simulink model "DriveSystemControl"  (R2023b)
settings: Solver=FixedStepAuto  StartTime=0.0  StopTime=Inf  FixedStep=0.001  RelTol=1e-3
PostLoadFcn:
  | if any(exist('dsrtsu_mdlpostloadfcn', 'file') ~= 0), dsrtsu_mdlpostloadfcn('Execute', bdroot); end
InitFcn:
  | , if any(exist('rtifpga_mdlclblib', 'file') ~= 0), rtifpga_mdlclblib('Init', bdroot); end,
  | , if any(exist('dsmpb_private', 'file') ~= 0), dsmpb_private('dsmpb_mdlclblib', 'Init', bdroot); end,
libraries: dsmpblib x2
(part 10 of 11)

== system DriveSystemControl/Bus Configuration (1) - Out/Manipulation/Virya Controller CAN File 08082024/WIP/CANChannel/PDUs/TCU04/sigMCU5_DriveMode/Feature Switch ==
  Feature Switch : Inport
  Term_sigMCU5_DriveMode Current Countdown Value : Terminator
  Term_sigMCU5_DriveMode Selected Feature : Terminator
  _Feature Switch_ : BusSelector  OutputSignals=sigMCU5_DriveMode Current Countdown Value,sigMCU5_DriveMode Selected Feature
  wires:
  Feature Switch/1 -> _Feature Switch_/1  "Feature Switch"
  _Feature Switch_/1 -> Term_sigMCU5_DriveMode Current Countdown Value/1  "<sigMCU5_DriveMode Current Countdown Value>"
  _Feature Switch_/2 -> Term_sigMCU5_DriveMode Selected Feature/1  "<sigMCU5_DriveMode Selected Feature>"

== system DriveSystemControl/Bus Configuration (1) - Out/Manipulation/Virya Controller CAN File 08082024/WIP/CANChannel/PDUs/TCU04/sigMCU5_Efficiency/Feature Switch ==
  Feature Switch : Inport
  Term_sigMCU5_Efficiency Current Countdown Value : Terminator
  Term_sigMCU5_Efficiency Selected Feature : Terminator
  _Feature Switch_ : BusSelector  OutputSignals=sigMCU5_Efficiency Current Countdown Value,sigMCU5_Efficiency Selected Feature
  wires:
  Feature Switch/1 -> _Feature Switch_/1  "Feature Switch"
  _Feature Switch_/1 -> Term_sigMCU5_Efficiency Current Countdown Value/1  "<sigMCU5_Efficiency Current Countdown Value>"
  _Feature Switch_/2 -> Term_sigMCU5_Efficiency Selected Feature/1  "<sigMCU5_Efficiency Selected Feature>"

== system DriveSystemControl/Bus Configuration (1) - Out/Manipulation/Virya Controller CAN File 08082024/WIP/CANChannel/PDUs/TCU04/sigMCU5_Hillhold/Feature Switch ==
  Feature Switch : Inport
  Term_sigMCU5_Hillhold Current Countdown Value : Terminator
  Term_sigMCU5_Hillhold Selected Feature : Terminator
  _Feature Switch_ : BusSelector  OutputSignals=sigMCU5_Hillhold Current Countdown Value,sigMCU5_Hillhold Selected Feature
  wires:
  Feature Switch/1 -> _Feature Switch_/1  "Feature Switch"
  _Feature Switch_/1 -> Term_sigMCU5_Hillhold Current Countdown Value/1  "<sigMCU5_Hillhold Current Countdown Value>"
  _Feature Switch_/2 -> Term_sigMCU5_Hillhold Selected Feature/1  "<sigMCU5_Hillhold Selected Feature>"

== system DriveSystemControl/Bus Configuration (1) - Out/Manipulation/Virya Controller CAN File 08082024/WIP/CANChannel/PDUs/TCU04/sigMCU5_RegenFlag/Feature Switch ==
  Feature Switch : Inport
  Term_sigMCU5_RegenFlag Current Countdown Value : Terminator
  Term_sigMCU5_RegenFlag Selected Feature : Terminator
  _Feature Switch_ : BusSelector  OutputSignals=sigMCU5_RegenFlag Current Countdown Value,sigMCU5_RegenFlag Selected Feature
  wires:
  Feature Switch/1 -> _Feature Switch_/1  "Feature Switch"
  _Feature Switch_/1 -> Term_sigMCU5_RegenFlag Current Countdown Value/1  "<sigMCU5_RegenFlag Current Countdown Value>"
  _Feature Switch_/2 -> Term_sigMCU5_RegenFlag Selected Feature/1  "<sigMCU5_RegenFlag Selected Feature>"

== system DriveSystemControl/Bus Configuration (1) - Out/Manipulation/Virya Controller CAN File 08082024/WIP/CANChannel/PDUs/TCU04/sigMCU5_Speed/Feature Switch ==
  Feature Switch : Inport
  Term_sigMCU5_Speed Current Countdown Value : Terminator
  Term_sigMCU5_Speed Selected Feature : Terminator
  _Feature Switch_ : BusSelector  OutputSignals=sigMCU5_Speed Current Countdown Value,sigMCU5_Speed Selected Feature
  wires:
  Feature Switch/1 -> _Feature Switch_/1  "Feature Switch"
  _Feature Switch_/1 -> Term_sigMCU5_Speed Current Countdown Value/1  "<sigMCU5_Speed Current Countdown Value>"
  _Feature Switch_/2 -> Term_sigMCU5_Speed Selected Feature/1  "<sigMCU5_Speed Selected Feature>"

== system DriveSystemControl/Bus Configuration (1) - Out/Manipulation/Virya Controller CAN File 08082024/WIP/CANChannel/PDUs/TCU05/sigMCU6_Odometer/Feature Switch ==
  Feature Switch : Inport
  Term_sigMCU6_Odometer Current Countdown Value : Terminator
  Term_sigMCU6_Odometer Selected Feature : Terminator
  _Feature Switch_ : BusSelector  OutputSignals=sigMCU6_Odometer Current Countdown Value,sigMCU6_Odometer Selected Feature
  wires:
  Feature Switch/1 -> _Feature Switch_/1  "Feature Switch"
  _Feature Switch_/1 -> Term_sigMCU6_Odometer Current Countdown Value/1  "<sigMCU6_Odometer Current Countdown Value>"
  _Feature Switch_/2 -> Term_sigMCU6_Odometer Selected Feature/1  "<sigMCU6_Odometer Selected Feature>"

== system DriveSystemControl/Bus Configuration (1) - Out/Simulated ECUs/Virya Controller CAN File 08082024/BMS/RX/PDUs/TCU04/sigMCU5_DriveMode/ISignal Value ==
  ISignal Value : Inport
  Term_sigMCU5_DriveMode Value : Terminator
  _ISignal Value_ : BusSelector  OutputSignals=sigMCU5_DriveMode Value
  wires:
  ISignal Value/1 -> _ISignal Value_/1  "ISignal Value"
  _ISignal Value_/1 -> Term_sigMCU5_DriveMode Value/1  "<sigMCU5_DriveMode Value>"

== system DriveSystemControl/Bus Configuration (1) - Out/Simulated ECUs/Virya Controller CAN File 08082024/BMS/RX/PDUs/TCU04/sigMCU5_Efficiency/ISignal Value ==
  ISignal Value : Inport
  Term_sigMCU5_Efficiency Value : Terminator
  _ISignal Value_ : BusSelector  OutputSignals=sigMCU5_Efficiency Value
  wires:
  ISignal Value/1 -> _ISignal Value_/1  "ISignal Value"
  _ISignal Value_/1 -> Term_sigMCU5_Efficiency Value/1  "<sigMCU5_Efficiency Value>"

== system DriveSystemControl/Bus Configuration (1) - Out/Simulated ECUs/Virya Controller CAN File 08082024/BMS/RX/PDUs/TCU04/sigMCU5_Hillhold/ISignal Value ==
  ISignal Value : Inport
  Term_sigMCU5_Hillhold Value : Terminator
  _ISignal Value_ : BusSelector  OutputSignals=sigMCU5_Hillhold Value
  wires:
  ISignal Value/1 -> _ISignal Value_/1  "ISignal Value"
  _ISignal Value_/1 -> Term_sigMCU5_Hillhold Value/1  "<sigMCU5_Hillhold Value>"

== system DriveSystemControl/Bus Configuration (1) - Out/Simulated ECUs/Virya Controller CAN File 08082024/BMS/RX/PDUs/TCU04/sigMCU5_RegenFlag/ISignal Value ==
  ISignal Value : Inport
  Term_sigMCU5_RegenFlag Value : Terminator
  _ISignal Value_ : BusSelector  OutputSignals=sigMCU5_RegenFlag Value
  wires:
  ISignal Value/1 -> _ISignal Value_/1  "ISignal Value"
  _ISignal Value_/1 -> Term_sigMCU5_RegenFlag Value/1  "<sigMCU5_RegenFlag Value>"

== system DriveSystemControl/Bus Configuration (1) - Out/Simulated ECUs/Virya Controller CAN File 08082024/BMS/RX/PDUs/TCU04/sigMCU5_Speed/ISignal Value ==
  ISignal Value : Inport
  Term_sigMCU5_Speed Value : Terminator
  _ISignal Value_ : BusSelector  OutputSignals=sigMCU5_Speed Value
  wires:
  ISignal Value/1 -> _ISignal Value_/1  "ISignal Value"
  _ISignal Value_/1 -> Term_sigMCU5_Speed Value/1  "<sigMCU5_Speed Value>"

== system DriveSystemControl/Bus Configuration (1) - Out/Simulated ECUs/Virya Controller CAN File 08082024/IPC/RX/PDUs/BMS01/sigBatteryMalfunctionLight/ISignal Value ==
  ISignal Value : Inport
  Term_sigBatteryMalfunctionLight Value : Terminator
  _ISignal Value_ : BusSelector  OutputSignals=sigBatteryMalfunctionLight Value
  wires:
  ISignal Value/1 -> _ISignal Value_/1  "ISignal Value"
  _ISignal Value_/1 -> Term_sigBatteryMalfunctionLight Value/1  "<sigBatteryMalfunctionLight Value>"

== system DriveSystemControl/Bus Configuration (1) - Out/Simulated ECUs/Virya Controller CAN File 08082024/IPC/RX/PDUs/BMS01/sigKeyOnIndicator/ISignal Value ==
  ISignal Value : Inport
  Term_sigKeyOnIndicator Value : Terminator
  _ISignal Value_ : BusSelector  OutputSignals=sigKeyOnIndicator Value
  wires:
  ISignal Value/1 -> _ISignal Value_/1  "ISignal Value"
  _ISignal Value_/1 -> Term_sigKeyOnIndicator Value/1  "<sigKeyOnIndicator Value>"

== system DriveSystemControl/Bus Configuration (1) - Out/Simulated ECUs/Virya Controller CAN File 08082024/IPC/RX/PDUs/BMS01/sigStateOfCharge/ISignal Value ==
  ISignal Value : Inport
  Term_sigStateOfCharge Value : Terminator
  _ISignal Value_ : BusSelector  OutputSignals=sigStateOfCharge Value
  wires:
  ISignal Value/1 -> _ISignal Value_/1  "ISignal Value"
  _ISignal Value_/1 -> Term_sigStateOfCharge Value/1  "<sigStateOfCharge Value>"

== system DriveSystemControl/Bus Configuration (1) - Out/Simulated ECUs/Virya Controller CAN File 08082024/IPC/RX/PDUs/TCU01/sigBrake/ISignal Value ==
  ISignal Value : Inport
  Term_sigBrake Value : Terminator
  _ISignal Value_ : BusSelector  OutputSignals=sigBrake Value
  wires:
  ISignal Value/1 -> _ISignal Value_/1  "ISignal Value"
  _ISignal Value_/1 -> Term_sigBrake Value/1  "<sigBrake Value>"

== system DriveSystemControl/Bus Configuration (1) - Out/Simulated ECUs/Virya Controller CAN File 08082024/IPC/RX/PDUs/TCU01/sigControllerTemperature/ISignal Value ==
  ISignal Value : Inport
  Term_sigControllerTemperature Value : Terminator
  _ISignal Value_ : BusSelector  OutputSignals=sigControllerTemperature Value
  wires:
  ISignal Value/1 -> _ISignal Value_/1  "ISignal Value"
  _ISignal Value_/1 -> Term_sigControllerTemperature Value/1  "<sigControllerTemperature Value>"

== system DriveSystemControl/Bus Configuration (1) - Out/Simulated ECUs/Virya Controller CAN File 08082024/IPC/RX/PDUs/TCU01/sigDriveMode/ISignal Value ==
  ISignal Value : Inport
  Term_sigDriveMode Value : Terminator
  _ISignal Value_ : BusSelector  OutputSignals=sigDriveMode Value
  wires:
  ISignal Value/1 -> _ISignal Value_/1  "ISignal Value"
  _ISignal Value_/1 -> Term_sigDriveMode Value/1  "<sigDriveMode Value>"

== system DriveSystemControl/Bus Configuration (1) - Out/Simulated ECUs/Virya Controller CAN File 08082024/IPC/RX/PDUs/TCU01/sigMotorTemperature/ISignal Value ==
  ISignal Value : Inport
  Term_sigMotorTemperature Value : Terminator
  _ISignal Value_ : BusSelector  OutputSignals=sigMotorTemperature Value
  wires:
  ISignal Value/1 -> _ISignal Value_/1  "ISignal Value"
  _ISignal Value_/1 -> Term_sigMotorTemperature Value/1  "<sigMotorTemperature Value>"

== system DriveSystemControl/Bus Configuration (1) - Out/Simulated ECUs/Virya Controller CAN File 08082024/IPC/RX/PDUs/TCU01/sigRMSCurrent/ISignal Value ==
  ISignal Value : Inport
  Term_sigRMSCurrent Value : Terminator
  _ISignal Value_ : BusSelector  OutputSignals=sigRMSCurrent Value
  wires:
  ISignal Value/1 -> _ISignal Value_/1  "ISignal Value"
  _ISignal Value_/1 -> Term_sigRMSCurrent Value/1  "<sigRMSCurrent Value>"

== system DriveSystemControl/Bus Configuration (1) - Out/Simulated ECUs/Virya Controller CAN File 08082024/IPC/RX/PDUs/TCU01/sigSpeed/ISignal Value ==
  ISignal Value : Inport
  Term_sigSpeed Value : Terminator
  _ISignal Value_ : BusSelector  OutputSignals=sigSpeed Value
  wires:
  ISignal Value/1 -> _ISignal Value_/1  "ISignal Value"
  _ISignal Value_/1 -> Term_sigSpeed Value/1  "<sigSpeed Value>"

== system DriveSystemControl/Bus Configuration (1) - Out/Simulated ECUs/Virya Controller CAN File 08082024/IPC/RX/PDUs/TCU01/sigThrottle/ISignal Value ==
  ISignal Value : Inport
  Term_sigThrottle Value : Terminator
  _ISignal Value_ : BusSelector  OutputSignals=sigThrottle Value
  wires:
  ISignal Value/1 -> _ISignal Value_/1  "ISignal Value"
  _ISignal Value_/1 -> Term_sigThrottle Value/1  "<sigThrottle Value>"

== system DriveSystemControl/Bus Configuration (1) - Out/Simulated ECUs/Virya Controller CAN File 08082024/IPC/RX/PDUs/TCU03/Controller_CompleteFaults/ISignal Value ==
  ISignal Value : Inport
  Term_Controller_CompleteFaults Value : Terminator
  _ISignal Value_ : BusSelector  OutputSignals=Controller_CompleteFaults Value
  wires:
  ISignal Value/1 -> _ISignal Value_/1  "ISignal Value"
  _ISignal Value_/1 -> Term_Controller_CompleteFaults Value/1  "<Controller_CompleteFaults Value>"

== system DriveSystemControl/Bus Configuration (1) - Out/Simulated ECUs/Virya Controller CAN File 08082024/IPC/RX/PDUs/TCU03/sig5VSupplyFailure/ISignal Value ==
  ISignal Value : Inport
  Term_sig5VSupplyFailure Value : Terminator
  _ISignal Value_ : BusSelector  OutputSignals=sig5VSupplyFailure Value
  wires:
  ISignal Value/1 -> _ISignal Value_/1  "ISignal Value"
  _ISignal Value_/1 -> Term_sig5VSupplyFailure Value/1  "<sig5VSupplyFailure Value>"

== system DriveSystemControl/Bus Configuration (1) - Out/Simulated ECUs/Virya Controller CAN File 08082024/IPC/RX/PDUs/TCU03/sigBPosOvervoltageCutback/ISignal Value ==
  ISignal Value : Inport
  Term_sigBPosOvervoltageCutback Value : Terminator
  _ISignal Value_ : BusSelector  OutputSignals=sigBPosOvervoltageCutback Value
  wires:
  ISignal Value/1 -> _ISignal Value_/1  "ISignal Value"
  _ISignal Value_/1 -> Term_sigBPosOvervoltageCutback Value/1  "<sigBPosOvervoltageCutback Value>"

== system DriveSystemControl/Bus Configuration (1) - Out/Simulated ECUs/Virya Controller CAN File 08082024/IPC/RX/PDUs/TCU03/sigBPosUndervoltageCutback/ISignal Value ==
  ISignal Value : Inport
  Term_sigBPosUndervoltageCutback Value : Terminator
  _ISignal Value_ : BusSelector  OutputSignals=sigBPosUndervoltageCutback Value
  wires:
  ISignal Value/1 -> _ISignal Value_/1  "ISignal Value"
  _ISignal Value_/1 -> Term_sigBPosUndervoltageCutback Value/1  "<sigBPosUndervoltageCutback Value>"

== system DriveSystemControl/Bus Configuration (1) - Out/Simulated ECUs/Virya Controller CAN File 08082024/IPC/RX/PDUs/TCU03/sigBadCalibration/ISignal Value ==
  ISignal Value : Inport
  Term_sigBadCalibration Value : Terminator
  _ISignal Value_ : BusSelector  OutputSignals=sigBadCalibration Value
  wires:
  ISignal Value/1 -> _ISignal Value_/1  "ISignal Value"
  _ISignal Value_/1 -> Term_sigBadCalibration Value/1  "<sigBadCalibration Value>"

== system DriveSystemControl/Bus Configuration (1) - Out/Simulated ECUs/Virya Controller CAN File 08082024/IPC/RX/PDUs/TCU03/sigBrakeWiperHigh/ISignal Value ==
  ISignal Value : Inport
  Term_sigBrakeWiperHigh Value : Terminator
  _ISignal Value_ : BusSelector  OutputSignals=sigBrakeWiperHigh Value
  wires:
  ISignal Value/1 -> _ISignal Value_/1  "ISignal Value"
  _ISignal Value_/1 -> Term_sigBrakeWiperHigh Value/1  "<sigBrakeWiperHigh Value>"

== system DriveSystemControl/Bus Configuration (1) - Out/Simulated ECUs/Virya Controller CAN File 08082024/IPC/RX/PDUs/TCU03/sigBrakeWiperLow/ISignal Value ==
  ISignal Value : Inport
  Term_sigBrakeWiperLow Value : Terminator
  _ISignal Value_ : BusSelector  OutputSignals=sigBrakeWiperLow Value
  wires:
  ISignal Value/1 -> _ISignal Value_/1  "ISignal Value"
  _ISignal Value_/1 -> Term_sigBrakeWiperLow Value/1  "<sigBrakeWiperLow Value>"

== system DriveSystemControl/Bus Configuration (1) - Out/Simulated ECUs/Virya Controller CAN File 08082024/IPC/RX/PDUs/TCU03/sigCoil2DriverOpenShort/ISignal Value ==
  ISignal Value : Inport
  Term_sigCoil2DriverOpenShort Value : Terminator
  _ISignal Value_ : BusSelector  OutputSignals=sigCoil2DriverOpenShort Value
  wires:
  ISignal Value/1 -> _ISignal Value_/1  "ISignal Value"
  _ISignal Value_/1 -> Term_sigCoil2DriverOpenShort Value/1  "<sigCoil2DriverOpenShort Value>"

== system DriveSystemControl/Bus Configuration (1) - Out/Simulated ECUs/Virya Controller CAN File 08082024/IPC/RX/PDUs/TCU03/sigCoil3DriverOpenShort/ISignal Value ==
  ISignal Value : Inport
  Term_sigCoil3DriverOpenShort Value : Terminator
  _ISignal Value_ : BusSelector  OutputSignals=sigCoil3DriverOpenShort Value
  wires:
  ISignal Value/1 -> _ISignal Value_/1  "ISignal Value"
  _ISignal Value_/1 -> Term_sigCoil3DriverOpenShort Value/1  "<sigCoil3DriverOpenShort Value>"

== system DriveSystemControl/Bus Configuration (1) - Out/Simulated ECUs/Virya Controller CAN File 08082024/IPC/RX/PDUs/TCU03/sigCoil4DriverOpenShort/ISignal Value ==
  ISignal Value : Inport
  Term_sigCoil4DriverOpenShort Value : Terminator
  _ISignal Value_ : BusSelector  OutputSignals=sigCoil4DriverOpenShort Value
  wires:
  ISignal Value/1 -> _ISignal Value_/1  "ISignal Value"
  _ISignal Value_/1 -> Term_sigCoil4DriverOpenShort Value/1  "<sigCoil4DriverOpenShort Value>"

== system DriveSystemControl/Bus Configuration (1) - Out/Simulated ECUs/Virya Controller CAN File 08082024/IPC/RX/PDUs/TCU03/sigControllerCommonFault/ISignal Value ==
  ISignal Value : Inport
  Term_sigControllerCommonFault Value : Terminator
  _ISignal Value_ : BusSelector  OutputSignals=sigControllerCommonFault Value
  wires:
  ISignal Value/1 -> _ISignal Value_/1  "ISignal Value"
  _ISignal Value_/1 -> Term_sigControllerCommonFault Value/1  "<sigControllerCommonFault Value>"

== system DriveSystemControl/Bus Configuration (1) - Out/Simulated ECUs/Virya Controller CAN File 08082024/IPC/RX/PDUs/TCU03/sigControllerOverCurrent/ISignal Value ==
  ISignal Value : Inport
  Term_sigControllerOverCurrent Value : Terminator
  _ISignal Value_ : BusSelector  OutputSignals=sigControllerOverCurrent Value
  wires:
  ISignal Value/1 -> _ISignal Value_/1  "ISignal Value"
  _ISignal Value_/1 -> Term_sigControllerOverCurrent Value/1  "<sigControllerOverCurrent Value>"

== system DriveSystemControl/Bus Configuration (1) - Out/Simulated ECUs/Virya Controller CAN File 08082024/IPC/RX/PDUs/TCU03/sigControllerOvertempCutback/ISignal Value ==
  ISignal Value : Inport
  Term_sigControllerOvertempCutback Value : Terminator
  _ISignal Value_ : BusSelector  OutputSignals=sigControllerOvertempCutback Value
  wires:
  ISignal Value/1 -> _ISignal Value_/1  "ISignal Value"
  _ISignal Value_/1 -> Term_sigControllerOvertempCutback Value/1  "<sigControllerOvertempCutback Value>"

== system DriveSystemControl/Bus Configuration (1) - Out/Simulated ECUs/Virya Controller CAN File 08082024/IPC/RX/PDUs/TCU03/sigControllerSevereOvertemp/ISignal Value ==
  ISignal Value : Inport
  Term_sigControllerSevereOvertemp Value : Terminator
  _ISignal Value_ : BusSelector  OutputSignals=sigControllerSevereOvertemp Value
  wires:
  ISignal Value/1 -> _ISignal Value_/1  "ISignal Value"
  _ISignal Value_/1 -> Term_sigControllerSevereOvertemp Value/1  "<sigControllerSevereOvertemp Value>"

== system DriveSystemControl/Bus Configuration (1) - Out/Simulated ECUs/Virya Controller CAN File 08082024/IPC/RX/PDUs/TCU03/sigControllerSevereUndertemp/ISignal Value ==
  ISignal Value : Inport
  Term_sigControllerSevereUndertemp Value : Terminator
  _ISignal Value_ : BusSelector  OutputSignals=sigControllerSevereUndertemp Value
  wires:
  ISignal Value/1 -> _ISignal Value_/1  "ISignal Value"
  _ISignal Value_/1 -> Term_sigControllerSevereUndertemp Value/1  "<sigControllerSevereUndertemp Value>"

== system DriveSystemControl/Bus Configuration (1) - Out/Simulated ECUs/Virya Controller CAN File 08082024/IPC/RX/PDUs/TCU03/sigCurrentSensorFault/ISignal Value ==
  ISignal Value : Inport
  Term_sigCurrentSensorFault Value : Terminator
  _ISignal Value_ : BusSelector  OutputSignals=sigCurrentSensorFault Value
  wires:
  ISignal Value/1 -> _ISignal Value_/1  "ISignal Value"
  _ISignal Value_/1 -> Term_sigCurrentSensorFault Value/1  "<sigCurrentSensorFault Value>"

== system DriveSystemControl/Bus Configuration (1) - Out/Simulated ECUs/Virya Controller CAN File 08082024/IPC/RX/PDUs/TCU03/sigEEPROMFailure/ISignal Value ==
  ISignal Value : Inport
  Term_sigEEPROMFailure Value : Terminator
  _ISignal Value_ : BusSelector  OutputSignals=sigEEPROMFailure Value
  wires:
  ISignal Value/1 -> _ISignal Value_/1  "ISignal Value"
  _ISignal Value_/1 -> Term_sigEEPROMFailure Value/1  "<sigEEPROMFailure Value>"

== system DriveSystemControl/Bus Configuration (1) - Out/Simulated ECUs/Virya Controller CAN File 08082024/IPC/RX/PDUs/TCU03/sigHighPedalDisable/ISignal Value ==
  ISignal Value : Inport
  Term_sigHighPedalDisable Value : Terminator
  _ISignal Value_ : BusSelector  OutputSignals=sigHighPedalDisable Value
  wires:
  ISignal Value/1 -> _ISignal Value_/1  "ISignal Value"
  _ISignal Value_/1 -> Term_sigHighPedalDisable Value/1  "<sigHighPedalDisable Value>"

== system DriveSystemControl/Bus Configuration (1) - Out/Simulated ECUs/Virya Controller CAN File 08082024/IPC/RX/PDUs/TCU03/sigInsulationResistanceLow/ISignal Value ==
  ISignal Value : Inport
  Term_sigInsulationResistanceLow Value : Terminator
  _ISignal Value_ : BusSelector  OutputSignals=sigInsulationResistanceLow Value
  wires:
  ISignal Value/1 -> _ISignal Value_/1  "ISignal Value"
  _ISignal Value_/1 -> Term_sigInsulationResistanceLow Value/1  "<sigInsulationResistanceLow Value>"

== system DriveSystemControl/Bus Configuration (1) - Out/Simulated ECUs/Virya Controller CAN File 08082024/IPC/RX/PDUs/TCU03/sigMainContactorWelded/ISignal Value ==
  ISignal Value : Inport
  Term_sigMainContactorWelded Value : Terminator
  _ISignal Value_ : BusSelector  OutputSignals=sigMainContactorWelded Value
  wires:
  ISignal Value/1 -> _ISignal Value_/1  "ISignal Value"
  _ISignal Value_/1 -> Term_sigMainContactorWelded Value/1  "<sigMainContactorWelded Value>"

== system DriveSystemControl/Bus Configuration (1) - Out/Simulated ECUs/Virya Controller CAN File 08082024/IPC/RX/PDUs/TCU03/sigMainContactordidnotClose/ISignal Value ==
  ISignal Value : Inport
  Term_sigMainContactordidnotClose Value : Terminator
  _ISignal Value_ : BusSelector  OutputSignals=sigMainContactordidnotClose Value
  wires:
  ISignal Value/1 -> _ISignal Value_/1  "ISignal Value"
  _ISignal Value_/1 -> Term_sigMainContactordidnotClose Value/1  "<sigMainContactordidnotClose Value>"

== system DriveSystemControl/Bus Configuration (1) - Out/Simulated ECUs/Virya Controller CAN File 08082024/IPC/RX/PDUs/TCU03/sigMainOpenShort/ISignal Value ==
  ISignal Value : Inport
  Term_sigMainOpenShort Value : Terminator
  _ISignal Value_ : BusSelector  OutputSignals=sigMainOpenShort Value
  wires:
  ISignal Value/1 -> _ISignal Value_/1  "ISignal Value"
  _ISignal Value_/1 -> Term_sigMainOpenShort Value/1  "<sigMainOpenShort Value>"

== system DriveSystemControl/Bus Configuration (1) - Out/Simulated ECUs/Virya Controller CAN File 08082024/IPC/RX/PDUs/TCU03/sigMotorCharacterization/ISignal Value ==
  ISignal Value : Inport
  Term_sigMotorCharacterization Value : Terminator
  _ISignal Value_ : BusSelector  OutputSignals=sigMotorCharacterization Value
  wires:
  ISignal Value/1 -> _ISignal Value_/1  "ISignal Value"
  _ISignal Value_/1 -> Term_sigMotorCharacterization Value/1  "<sigMotorCharacterization Value>"

== system DriveSystemControl/Bus Configuration (1) - Out/Simulated ECUs/Virya Controller CAN File 08082024/IPC/RX/PDUs/TCU03/sigMotorPhaseOpen/ISignal Value ==
  ISignal Value : Inport
  Term_sigMotorPhaseOpen Value : Terminator
  _ISignal Value_ : BusSelector  OutputSignals=sigMotorPhaseOpen Value
  wires:
  ISignal Value/1 -> _ISignal Value_/1  "ISignal Value"
  _ISignal Value_/1 -> Term_sigMotorPhaseOpen Value/1  "<sigMotorPhaseOpen Value>"

== system DriveSystemControl/Bus Configuration (1) - Out/Simulated ECUs/Virya Controller CAN File 08082024/IPC/RX/PDUs/TCU03/sigMotorTempHotCutback/ISignal Value ==
  ISignal Value : Inport
  Term_sigMotorTempHotCutback Value : Terminator
  _ISignal Value_ : BusSelector  OutputSignals=sigMotorTempHotCutback Value
  wires:
  ISignal Value/1 -> _ISignal Value_/1  "ISignal Value"
  _ISignal Value_/1 -> Term_sigMotorTempHotCutback Value/1  "<sigMotorTempHotCutback Value>"

== system DriveSystemControl/Bus Configuration (1) - Out/Simulated ECUs/Virya Controller CAN File 08082024/IPC/RX/PDUs/TCU03/sigMotorTempSensorFault/ISignal Value ==
  ISignal Value : Inport
  Term_sigMotorTempSensorFault Value : Terminator
  _ISignal Value_ : BusSelector  OutputSignals=sigMotorTempSensorFault Value
  wires:
  ISignal Value/1 -> _ISignal Value_/1  "ISignal Value"
  _ISignal Value_/1 -> Term_sigMotorTempSensorFault Value/1  "<sigMotorTempSensorFault Value>"

== system DriveSystemControl/Bus Configuration (1) - Out/Simulated ECUs/Virya Controller CAN File 08082024/IPC/RX/PDUs/TCU03/sigOEM_BatterySTOPSignal/ISignal Value ==
  ISignal Value : Inport
  Term_sigOEM_BatterySTOPSignal Value : Terminator
  _ISignal Value_ : BusSelector  OutputSignals=sigOEM_BatterySTOPSignal Value
  wires:
  ISignal Value/1 -> _ISignal Value_/1  "ISignal Value"
  _ISignal Value_/1 -> Term_sigOEM_BatterySTOPSignal Value/1  "<sigOEM_BatterySTOPSignal Value>"

== system DriveSystemControl/Bus Configuration (1) - Out/Simulated ECUs/Virya Controller CAN File 08082024/IPC/RX/PDUs/TCU03/sigOEM_NoBatteryCAN/ISignal Value ==
  ISignal Value : Inport
  Term_sigOEM_NoBatteryCAN Value : Terminator
  _ISignal Value_ : BusSelector  OutputSignals=sigOEM_NoBatteryCAN Value
  wires:
  ISignal Value/1 -> _ISignal Value_/1  "ISignal Value"
  _ISignal Value_/1 -> Term_sigOEM_NoBatteryCAN Value/1  "<sigOEM_NoBatteryCAN Value>"

== system DriveSystemControl/Bus Configuration (1) - Out/Simulated ECUs/Virya Controller CAN File 08082024/IPC/RX/PDUs/TCU03/sigOSGeneral/ISignal Value ==
  ISignal Value : Inport
  Term_sigOSGeneral Value : Terminator
  _ISignal Value_ : BusSelector  OutputSignals=sigOSGeneral Value
  wires:
  ISignal Value/1 -> _ISignal Value_/1  "ISignal Value"
  _ISignal Value_/1 -> Term_sigOSGeneral Value/1  "<sigOSGeneral Value>"

== system DriveSystemControl/Bus Configuration (1) - Out/Simulated ECUs/Virya Controller CAN File 08082024/IPC/RX/PDUs/TCU03/sigPMACCommissioningNeeded/ISignal Value ==
  ISignal Value : Inport
  Term_sigPMACCommissioningNeeded Value : Terminator
  _ISignal Value_ : BusSelector  OutputSignals=sigPMACCommissioningNeeded Value
  wires:
  ISignal Value/1 -> _ISignal Value_/1  "ISignal Value"
  _ISignal Value_/1 -> Term_sigPMACCommissioningNeeded Value/1  "<sigPMACCommissioningNeeded Value>"

== system DriveSystemControl/Bus Configuration (1) - Out/Simulated ECUs/Virya Controller CAN File 08082024/IPC/RX/PDUs/TCU03/sigParameterChangeFault/ISignal Value ==
  ISignal Value : Inport
  Term_sigParameterChangeFault Value : Terminator
  _ISignal Value_ : BusSelector  OutputSignals=sigParameterChangeFault Value
  wires:
  ISignal Value/1 -> _ISignal Value_/1  "ISignal Value"
  _ISignal Value_/1 -> Term_sigParameterChangeFault Value/1  "<sigParameterChangeFault Value>"

== system DriveSystemControl/Bus Configuration (1) - Out/Simulated ECUs/Virya Controller CAN File 08082024/IPC/RX/PDUs/TCU03/sigPhasePWMMismatch/ISignal Value ==
  ISignal Value : Inport
  Term_sigPhasePWMMismatch Value : Terminator
  _ISignal Value_ : BusSelector  OutputSignals=sigPhasePWMMismatch Value
  wires:
  ISignal Value/1 -> _ISignal Value_/1  "ISignal Value"
  _ISignal Value_/1 -> Term_sigPhasePWMMismatch Value/1  "<sigPhasePWMMismatch Value>"

== system DriveSystemControl/Bus Configuration (1) - Out/Simulated ECUs/Virya Controller CAN File 08082024/IPC/RX/PDUs/TCU03/sigPrechargeFailed/ISignal Value ==
  ISignal Value : Inport
  Term_sigPrechargeFailed Value : Terminator
  _ISignal Value_ : BusSelector  OutputSignals=sigPrechargeFailed Value
  wires:
  ISignal Value/1 -> _ISignal Value_/1  "ISignal Value"
  _ISignal Value_/1 -> Term_sigPrechargeFailed Value/1  "<sigPrechargeFailed Value>"

== system DriveSystemControl/Bus Configuration (1) - Out/Simulated ECUs/Virya Controller CAN File 08082024/IPC/RX/PDUs/TCU03/sigSevereBPosOvervoltage/ISignal Value ==
  ISignal Value : Inport
  Term_sigSevereBPosOvervoltage Value : Terminator
  _ISignal Value_ : BusSelector  OutputSignals=sigSevereBPosOvervoltage Value
  wires:
  ISignal Value/1 -> _ISignal Value_/1  "ISignal Value"
  _ISignal Value_/1 -> Term_sigSevereBPosOvervoltage Value/1  "<sigSevereBPosOvervoltage Value>"

== system DriveSystemControl/Bus Configuration (1) - Out/Simulated ECUs/Virya Controller CAN File 08082024/IPC/RX/PDUs/TCU03/sigSevereBPosUndervoltage/ISignal Value ==
  ISignal Value : Inport
  Term_sigSevereBPosUndervoltage Value : Terminator
  _ISignal Value_ : BusSelector  OutputSignals=sigSevereBPosUndervoltage Value
  wires:
  ISignal Value/1 -> _ISignal Value_/1  "ISignal Value"
  _ISignal Value_/1 -> Term_sigSevereBPosUndervoltage Value/1  "<sigSevereBPosUndervoltage Value>"

== system DriveSystemControl/Bus Configuration (1) - Out/Simulated ECUs/Virya Controller CAN File 08082024/IPC/RX/PDUs/TCU03/sigSevereKSIOvervoltage/ISignal Value ==
  ISignal Value : Inport
  Term_sigSevereKSIOvervoltage Value : Terminator
  _ISignal Value_ : BusSelector  OutputSignals=sigSevereKSIOvervoltage Value
  wires:
  ISignal Value/1 -> _ISignal Value_/1  "ISignal Value"
  _ISignal Value_/1 -> Term_sigSevereKSIOvervoltage Value/1  "<sigSevereKSIOvervoltage Value>"

== system DriveSystemControl/Bus Configuration (1) - Out/Simulated ECUs/Virya Controller CAN File 08082024/IPC/RX/PDUs/TCU03/sigSevereKSIUndervoltage/ISignal Value ==
  ISignal Value : Inport
  Term_sigSevereKSIUndervoltage Value : Terminator
  _ISignal Value_ : BusSelector  OutputSignals=sigSevereKSIUndervoltage Value
  wires:
  ISignal Value/1 -> _ISignal Value_/1  "ISignal Value"
  _ISignal Value_/1 -> Term_sigSevereKSIUndervoltage Value/1  "<sigSevereKSIUndervoltage Value>"

== system DriveSystemControl/Bus Configuration (1) - Out/Simulated ECUs/Virya Controller CAN File 08082024/IPC/RX/PDUs/TCU03/sigSinCosMisalignment/ISignal Value ==
  ISignal Value : Inport
  Term_sigSinCosMisalignment Value : Terminator
  _ISignal Value_ : BusSelector  OutputSignals=sigSinCosMisalignment Value
  wires:
  ISignal Value/1 -> _ISignal Value_/1  "ISignal Value"
  _ISignal Value_/1 -> Term_sigSinCosMisalignment Value/1  "<sigSinCosMisalignment Value>"

== system DriveSystemControl/Bus Configuration (1) - Out/Simulated ECUs/Virya Controller CAN File 08082024/IPC/RX/PDUs/TCU03/sigSinCosSensorFault/ISignal Value ==
  ISignal Value : Inport
  Term_sigSinCosSensorFault Value : Terminator
  _ISignal Value_ : BusSelector  OutputSignals=sigSinCosSensorFault Value
  wires:
  ISignal Value/1 -> _ISignal Value_/1  "ISignal Value"
  _ISignal Value_/1 -> Term_sigSinCosSensorFault Value/1  "<sigSinCosSensorFault Value>"

== system DriveSystemControl/Bus Configuration (1) - Out/Simulated ECUs/Virya Controller CAN File 08082024/IPC/RX/PDUs/TCU03/sigStallDetected/ISignal Value ==
  ISignal Value : Inport
  Term_sigStallDetected Value : Terminator
  _ISignal Value_ : BusSelector  OutputSignals=sigStallDetected Value
  wires:
  ISignal Value/1 -> _ISignal Value_/1  "ISignal Value"
  _ISignal Value_/1 -> Term_sigStallDetected Value/1  "<sigStallDetected Value>"

== system DriveSystemControl/Bus Configuration (1) - Out/Simulated ECUs/Virya Controller CAN File 08082024/IPC/RX/PDUs/TCU03/sigSupervisorFault/ISignal Value ==
  ISignal Value : Inport
  Term_sigSupervisorFault Value : Terminator
  _ISignal Value_ : BusSelector  OutputSignals=sigSupervisorFault Value
  wires:
  ISignal Value/1 -> _ISignal Value_/1  "ISignal Value"
  _ISignal Value_/1 -> Term_sigSupervisorFault Value/1  "<sigSupervisorFault Value>"

== system DriveSystemControl/Bus Configuration (1) - Out/Simulated ECUs/Virya Controller CAN File 08082024/IPC/RX/PDUs/TCU03/sigThrottlewiperHigh/ISignal Value ==
  ISignal Value : Inport
  Term_sigThrottlewiperHigh Value : Terminator
  _ISignal Value_ : BusSelector  OutputSignals=sigThrottlewiperHigh Value
  wires:
  ISignal Value/1 -> _ISignal Value_/1  "ISignal Value"
  _ISignal Value_/1 -> Term_sigThrottlewiperHigh Value/1  "<sigThrottlewiperHigh Value>"

== system DriveSystemControl/Bus Configuration (1) - Out/Simulated ECUs/Virya Controller CAN File 08082024/IPC/RX/PDUs/TCU03/sigThrottlewiperLow/ISignal Value ==
  ISignal Value : Inport
  Term_sigThrottlewiperLow Value : Terminator
  _ISignal Value_ : BusSelector  OutputSignals=sigThrottlewiperLow Value
  wires:
  ISignal Value/1 -> _ISignal Value_/1  "ISignal Value"
  _ISignal Value_/1 -> Term_sigThrottlewiperLow Value/1  "<sigThrottlewiperLow Value>"

== system DriveSystemControl/Bus Configuration (1) - Out/Simulated ECUs/Virya Controller CAN File 08082024/IPC/RX/PDUs/TCU03/sigVCLRunTimeError/ISignal Value ==
  ISignal Value : Inport
  Term_sigVCLRunTimeError Value : Terminator
  _ISignal Value_ : BusSelector  OutputSignals=sigVCLRunTimeError Value
  wires:
  ISignal Value/1 -> _ISignal Value_/1  "ISignal Value"
  _ISignal Value_/1 -> Term_sigVCLRunTimeError Value/1  "<sigVCLRunTimeError Value>"

== system DriveSystemControl/Bus Configuration (1) - Out/Simulated ECUs/Virya Controller CAN File 08082024/IPC/RX/PDUs/TCU04/sigMCU5_DriveMode/ISignal Value ==
  ISignal Value : Inport
  Term_sigMCU5_DriveMode Value : Terminator
  _ISignal Value_ : BusSelector  OutputSignals=sigMCU5_DriveMode Value
  wires:
  ISignal Value/1 -> _ISignal Value_/1  "ISignal Value"
  _ISignal Value_/1 -> Term_sigMCU5_DriveMode Value/1  "<sigMCU5_DriveMode Value>"

== system DriveSystemControl/Bus Configuration (1) - Out/Simulated ECUs/Virya Controller CAN File 08082024/IPC/RX/PDUs/TCU04/sigMCU5_Efficiency/ISignal Value ==
  ISignal Value : Inport
  Term_sigMCU5_Efficiency Value : Terminator
  _ISignal Value_ : BusSelector  OutputSignals=sigMCU5_Efficiency Value
  wires:
  ISignal Value/1 -> _ISignal Value_/1  "ISignal Value"
  _ISignal Value_/1 -> Term_sigMCU5_Efficiency Value/1  "<sigMCU5_Efficiency Value>"

== system DriveSystemControl/Bus Configuration (1) - Out/Simulated ECUs/Virya Controller CAN File 08082024/IPC/RX/PDUs/TCU04/sigMCU5_Hillhold/ISignal Value ==
  ISignal Value : Inport
  Term_sigMCU5_Hillhold Value : Terminator
  _ISignal Value_ : BusSelector  OutputSignals=sigMCU5_Hillhold Value
  wires:
  ISignal Value/1 -> _ISignal Value_/1  "ISignal Value"
  _ISignal Value_/1 -> Term_sigMCU5_Hillhold Value/1  "<sigMCU5_Hillhold Value>"

== system DriveSystemControl/Bus Configuration (1) - Out/Simulated ECUs/Virya Controller CAN File 08082024/IPC/RX/PDUs/TCU04/sigMCU5_RegenFlag/ISignal Value ==
  ISignal Value : Inport
  Term_sigMCU5_RegenFlag Value : Terminator
  _ISignal Value_ : BusSelector  OutputSignals=sigMCU5_RegenFlag Value
  wires:
  ISignal Value/1 -> _ISignal Value_/1  "ISignal Value"
  _ISignal Value_/1 -> Term_sigMCU5_RegenFlag Value/1  "<sigMCU5_RegenFlag Value>"

== system DriveSystemControl/Bus Configuration (1) - Out/Simulated ECUs/Virya Controller CAN File 08082024/IPC/RX/PDUs/TCU04/sigMCU5_Speed/ISignal Value ==
  ISignal Value : Inport
  Term_sigMCU5_Speed Value : Terminator
  _ISignal Value_ : BusSelector  OutputSignals=sigMCU5_Speed Value
  wires:
  ISignal Value/1 -> _ISignal Value_/1  "ISignal Value"
  _ISignal Value_/1 -> Term_sigMCU5_Speed Value/1  "<sigMCU5_Speed Value>"

== system DriveSystemControl/Bus Configuration (1) - Out/Simulated ECUs/Virya Controller CAN File 08082024/IPC/RX/PDUs/TCU05/sigMCU6_Odometer/ISignal Value ==
  ISignal Value : Inport
  Term_sigMCU6_Odometer Value : Terminator
  _ISignal Value_ : BusSelector  OutputSignals=sigMCU6_Odometer Value
  wires:
  ISignal Value/1 -> _ISignal Value_/1  "ISignal Value"
  _ISignal Value_/1 -> Term_sigMCU6_Odometer Value/1  "<sigMCU6_Odometer Value>"

== system DriveSystemControl/Bus Configuration (1) - Out/Simulated ECUs/Virya Controller CAN File 08082024/TCU/RX/PDUs/BMS02/sigBatteryCurrent/ISignal Value ==
  ISignal Value : Inport
  Term_sigBatteryCurrent Value : Terminator
  _ISignal Value_ : BusSelector  OutputSignals=sigBatteryCurrent Value
  wires:
  ISignal Value/1 -> _ISignal Value_/1  "ISignal Value"
  _ISignal Value_/1 -> Term_sigBatteryCurrent Value/1  "<sigBatteryCurrent Value>"

== system DriveSystemControl/Bus Configuration (1) - Out/Simulated ECUs/Virya Controller CAN File 08082024/TCU/RX/PDUs/BMS02/sigDriveCurrentLimit/ISignal Value ==
  ISignal Value : Inport
  Term_sigDriveCurrentLimit Value : Terminator
  _ISignal Value_ : BusSelector  OutputSignals=sigDriveCurrentLimit Value
  wires:
  ISignal Value/1 -> _ISignal Value_/1  "ISignal Value"
  _ISignal Value_/1 -> Term_sigDriveCurrentLimit Value/1  "<sigDriveCurrentLimit Value>"

== system DriveSystemControl/Bus Configuration (1) - Out/Simulated ECUs/Virya Controller CAN File 08082024/TCU/RX/PDUs/BMS02/sigRegenCurrentLimit/ISignal Value ==
  ISignal Value : Inport
  Term_sigRegenCurrentLimit Value : Terminator
  _ISignal Value_ : BusSelector  OutputSignals=sigRegenCurrentLimit Value
  wires:
  ISignal Value/1 -> _ISignal Value_/1  "ISignal Value"
  _ISignal Value_/1 -> Term_sigRegenCurrentLimit Value/1  "<sigRegenCurrentLimit Value>"

== system DriveSystemControl/Bus Configuration (1) - Out/Simulated ECUs/Virya Controller CAN File 08082024/TCU/RX/PDUs/BMS02/sigVehicleModeRequest/ISignal Value ==
  ISignal Value : Inport
  Term_sigVehicleModeRequest Value : Terminator
  _ISignal Value_ : BusSelector  OutputSignals=sigVehicleModeRequest Value
  wires:
  ISignal Value/1 -> _ISignal Value_/1  "ISignal Value"
  _ISignal Value_/1 -> Term_sigVehicleModeRequest Value/1  "<sigVehicleModeRequest Value>"

== system DriveSystemControl/Bus Configuration (1) - Out/Simulated ECUs/Virya Controller CAN File 08082024/Telematics/RX/PDUs/BMS01/sigBatteryMalfunctionLight/ISignal Value ==
  ISignal Value : Inport
  Term_sigBatteryMalfunctionLight Value : Terminator
  _ISignal Value_ : BusSelector  OutputSignals=sigBatteryMalfunctionLight Value
  wires:
  ISignal Value/1 -> _ISignal Value_/1  "ISignal Value"
  _ISignal Value_/1 -> Term_sigBatteryMalfunctionLight Value/1  "<sigBatteryMalfunctionLight Value>"

== system DriveSystemControl/Bus Configuration (1) - Out/Simulated ECUs/Virya Controller CAN File 08082024/Telematics/RX/PDUs/BMS01/sigKeyOnIndicator/ISignal Value ==
  ISignal Value : Inport
  Term_sigKeyOnIndicator Value : Terminator
  _ISignal Value_ : BusSelector  OutputSignals=sigKeyOnIndicator Value
  wires:
  ISignal Value/1 -> _ISignal Value_/1  "ISignal Value"
  _ISignal Value_/1 -> Term_sigKeyOnIndicator Value/1  "<sigKeyOnIndicator Value>"

== system DriveSystemControl/Bus Configuration (1) - Out/Simulated ECUs/Virya Controller CAN File 08082024/Telematics/RX/PDUs/BMS01/sigStateOfCharge/ISignal Value ==
  ISignal Value : Inport
  Term_sigStateOfCharge Value : Terminator
  _ISignal Value_ : BusSelector  OutputSignals=sigStateOfCharge Value
  wires:
  ISignal Value/1 -> _ISignal Value_/1  "ISignal Value"
  _ISignal Value_/1 -> Term_sigStateOfCharge Value/1  "<sigStateOfCharge Value>"

== system DriveSystemControl/Bus Configuration (1) - Out/Simulated ECUs/Virya Controller CAN File 08082024/Telematics/RX/PDUs/BMS02/sigBatteryCurrent/ISignal Value ==
  ISignal Value : Inport
  Term_sigBatteryCurrent Value : Terminator
  _ISignal Value_ : BusSelector  OutputSignals=sigBatteryCurrent Value
  wires:
  ISignal Value/1 -> _ISignal Value_/1  "ISignal Value"
  _ISignal Value_/1 -> Term_sigBatteryCurrent Value/1  "<sigBatteryCurrent Value>"

== system DriveSystemControl/Bus Configuration (1) - Out/Simulated ECUs/Virya Controller CAN File 08082024/Telematics/RX/PDUs/BMS02/sigDriveCurrentLimit/ISignal Value ==
  ISignal Value : Inport
  Term_sigDriveCurrentLimit Value : Terminator
  _ISignal Value_ : BusSelector  OutputSignals=sigDriveCurrentLimit Value
  wires:
  ISignal Value/1 -> _ISignal Value_/1  "ISignal Value"
  _ISignal Value_/1 -> Term_sigDriveCurrentLimit Value/1  "<sigDriveCurrentLimit Value>"

== system DriveSystemControl/Bus Configuration (1) - Out/Simulated ECUs/Virya Controller CAN File 08082024/Telematics/RX/PDUs/BMS02/sigRegenCurrentLimit/ISignal Value ==
  ISignal Value : Inport
  Term_sigRegenCurrentLimit Value : Terminator
  _ISignal Value_ : BusSelector  OutputSignals=sigRegenCurrentLimit Value
  wires:
  ISignal Value/1 -> _ISignal Value_/1  "ISignal Value"
  _ISignal Value_/1 -> Term_sigRegenCurrentLimit Value/1  "<sigRegenCurrentLimit Value>"

== system DriveSystemControl/Bus Configuration (1) - Out/Simulated ECUs/Virya Controller CAN File 08082024/Telematics/RX/PDUs/BMS02/sigVehicleModeRequest/ISignal Value ==
  ISignal Value : Inport
  Term_sigVehicleModeRequest Value : Terminator
  _ISignal Value_ : BusSelector  OutputSignals=sigVehicleModeRequest Value
  wires:
  ISignal Value/1 -> _ISignal Value_/1  "ISignal Value"
  _ISignal Value_/1 -> Term_sigVehicleModeRequest Value/1  "<sigVehicleModeRequest Value>"

== system DriveSystemControl/Bus Configuration (1) - Out/Simulated ECUs/Virya Controller CAN File 08082024/Telematics/RX/PDUs/TCU01/sigBrake/ISignal Value ==
  ISignal Value : Inport
  Term_sigBrake Value : Terminator
  _ISignal Value_ : BusSelector  OutputSignals=sigBrake Value
  wires:
  ISignal Value/1 -> _ISignal Value_/1  "ISignal Value"
  _ISignal Value_/1 -> Term_sigBrake Value/1  "<sigBrake Value>"

== system DriveSystemControl/Bus Configuration (1) - Out/Simulated ECUs/Virya Controller CAN File 08082024/Telematics/RX/PDUs/TCU01/sigControllerTemperature/ISignal Value ==
  ISignal Value : Inport
  Term_sigControllerTemperature Value : Terminator
  _ISignal Value_ : BusSelector  OutputSignals=sigControllerTemperature Value
  wires:
  ISignal Value/1 -> _ISignal Value_/1  "ISignal Value"
  _ISignal Value_/1 -> Term_sigControllerTemperature Value/1  "<sigControllerTemperature Value>"

== system DriveSystemControl/Bus Configuration (1) - Out/Simulated ECUs/Virya Controller CAN File 08082024/Telematics/RX/PDUs/TCU01/sigDriveMode/ISignal Value ==
  ISignal Value : Inport
  Term_sigDriveMode Value : Terminator
  _ISignal Value_ : BusSelector  OutputSignals=sigDriveMode Value
  wires:
  ISignal Value/1 -> _ISignal Value_/1  "ISignal Value"
  _ISignal Value_/1 -> Term_sigDriveMode Value/1  "<sigDriveMode Value>"

== system DriveSystemControl/Bus Configuration (1) - Out/Simulated ECUs/Virya Controller CAN File 08082024/Telematics/RX/PDUs/TCU01/sigMotorTemperature/ISignal Value ==
  ISignal Value : Inport
  Term_sigMotorTemperature Value : Terminator
  _ISignal Value_ : BusSelector  OutputSignals=sigMotorTemperature Value
  wires:
  ISignal Value/1 -> _ISignal Value_/1  "ISignal Value"
  _ISignal Value_/1 -> Term_sigMotorTemperature Value/1  "<sigMotorTemperature Value>"

== system DriveSystemControl/Bus Configuration (1) - Out/Simulated ECUs/Virya Controller CAN File 08082024/Telematics/RX/PDUs/TCU01/sigRMSCurrent/ISignal Value ==
  ISignal Value : Inport
  Term_sigRMSCurrent Value : Terminator
  _ISignal Value_ : BusSelector  OutputSignals=sigRMSCurrent Value
  wires:
  ISignal Value/1 -> _ISignal Value_/1  "ISignal Value"
  _ISignal Value_/1 -> Term_sigRMSCurrent Value/1  "<sigRMSCurrent Value>"

== system DriveSystemControl/Bus Configuration (1) - Out/Simulated ECUs/Virya Controller CAN File 08082024/Telematics/RX/PDUs/TCU01/sigSpeed/ISignal Value ==
  ISignal Value : Inport
  Term_sigSpeed Value : Terminator
  _ISignal Value_ : BusSelector  OutputSignals=sigSpeed Value
  wires:
  ISignal Value/1 -> _ISignal Value_/1  "ISignal Value"
  _ISignal Value_/1 -> Term_sigSpeed Value/1  "<sigSpeed Value>"

== system DriveSystemControl/Bus Configuration (1) - Out/Simulated ECUs/Virya Controller CAN File 08082024/Telematics/RX/PDUs/TCU01/sigThrottle/ISignal Value ==
  ISignal Value : Inport
  Term_sigThrottle Value : Terminator
  _ISignal Value_ : BusSelector  OutputSignals=sigThrottle Value
  wires:
  ISignal Value/1 -> _ISignal Value_/1  "ISignal Value"
  _ISignal Value_/1 -> Term_sigThrottle Value/1  "<sigThrottle Value>"

== system DriveSystemControl/Bus Configuration (1) - Out/Simulated ECUs/Virya Controller CAN File 08082024/Telematics/RX/PDUs/TCU02/sigCapacitorVoltage/ISignal Value ==
  ISignal Value : Inport
  Term_sigCapacitorVoltage Value : Terminator
  _ISignal Value_ : BusSelector  OutputSignals=sigCapacitorVoltage Value
  wires:
  ISignal Value/1 -> _ISignal Value_/1  "ISignal Value"
  _ISignal Value_/1 -> Term_sigCapacitorVoltage Value/1  "<sigCapacitorVoltage Value>"

== system DriveSystemControl/Bus Configuration (1) - Out/Simulated ECUs/Virya Controller CAN File 08082024/Telematics/RX/PDUs/TCU02/sigMotorRPM/ISignal Value ==
  ISignal Value : Inport
  Term_sigMotorRPM Value : Terminator
  _ISignal Value_ : BusSelector  OutputSignals=sigMotorRPM Value
  wires:
  ISignal Value/1 -> _ISignal Value_/1  "ISignal Value"
  _ISignal Value_/1 -> Term_sigMotorRPM Value/1  "<sigMotorRPM Value>"

== system DriveSystemControl/Bus Configuration (1) - Out/Simulated ECUs/Virya Controller CAN File 08082024/Telematics/RX/PDUs/TCU02/sigOdometer/ISignal Value ==
  ISignal Value : Inport
  Term_sigOdometer Value : Terminator
  _ISignal Value_ : BusSelector  OutputSignals=sigOdometer Value
  wires:
  ISignal Value/1 -> _ISignal Value_/1  "ISignal Value"
  _ISignal Value_/1 -> Term_sigOdometer Value/1  "<sigOdometer Value>"

== system DriveSystemControl/Bus Configuration (1) - Out/Simulated ECUs/Virya Controller CAN File 08082024/Telematics/RX/PDUs/TCU03/Controller_CompleteFaults/ISignal Value ==
  ISignal Value : Inport
  Term_Controller_CompleteFaults Value : Terminator
  _ISignal Value_ : BusSelector  OutputSignals=Controller_CompleteFaults Value
  wires:
  ISignal Value/1 -> _ISignal Value_/1  "ISignal Value"
  _ISignal Value_/1 -> Term_Controller_CompleteFaults Value/1  "<Controller_CompleteFaults Value>"

== system DriveSystemControl/Bus Configuration (1) - Out/Simulated ECUs/Virya Controller CAN File 08082024/Telematics/RX/PDUs/TCU03/sig5VSupplyFailure/ISignal Value ==
  ISignal Value : Inport
  Term_sig5VSupplyFailure Value : Terminator
  _ISignal Value_ : BusSelector  OutputSignals=sig5VSupplyFailure Value
  wires:
  ISignal Value/1 -> _ISignal Value_/1  "ISignal Value"
  _ISignal Value_/1 -> Term_sig5VSupplyFailure Value/1  "<sig5VSupplyFailure Value>"

== system DriveSystemControl/Bus Configuration (1) - Out/Simulated ECUs/Virya Controller CAN File 08082024/Telematics/RX/PDUs/TCU03/sigBPosOvervoltageCutback/ISignal Value ==
  ISignal Value : Inport
  Term_sigBPosOvervoltageCutback Value : Terminator
  _ISignal Value_ : BusSelector  OutputSignals=sigBPosOvervoltageCutback Value
  wires:
  ISignal Value/1 -> _ISignal Value_/1  "ISignal Value"
  _ISignal Value_/1 -> Term_sigBPosOvervoltageCutback Value/1  "<sigBPosOvervoltageCutback Value>"

== system DriveSystemControl/Bus Configuration (1) - Out/Simulated ECUs/Virya Controller CAN File 08082024/Telematics/RX/PDUs/TCU03/sigBPosUndervoltageCutback/ISignal Value ==
  ISignal Value : Inport
  Term_sigBPosUndervoltageCutback Value : Terminator
  _ISignal Value_ : BusSelector  OutputSignals=sigBPosUndervoltageCutback Value
  wires:
  ISignal Value/1 -> _ISignal Value_/1  "ISignal Value"
  _ISignal Value_/1 -> Term_sigBPosUndervoltageCutback Value/1  "<sigBPosUndervoltageCutback Value>"

== system DriveSystemControl/Bus Configuration (1) - Out/Simulated ECUs/Virya Controller CAN File 08082024/Telematics/RX/PDUs/TCU03/sigBadCalibration/ISignal Value ==
  ISignal Value : Inport
  Term_sigBadCalibration Value : Terminator
  _ISignal Value_ : BusSelector  OutputSignals=sigBadCalibration Value
  wires:
  ISignal Value/1 -> _ISignal Value_/1  "ISignal Value"
  _ISignal Value_/1 -> Term_sigBadCalibration Value/1  "<sigBadCalibration Value>"

== system DriveSystemControl/Bus Configuration (1) - Out/Simulated ECUs/Virya Controller CAN File 08082024/Telematics/RX/PDUs/TCU03/sigBrakeWiperHigh/ISignal Value ==
  ISignal Value : Inport
  Term_sigBrakeWiperHigh Value : Terminator
  _ISignal Value_ : BusSelector  OutputSignals=sigBrakeWiperHigh Value
  wires:
  ISignal Value/1 -> _ISignal Value_/1  "ISignal Value"
  _ISignal Value_/1 -> Term_sigBrakeWiperHigh Value/1  "<sigBrakeWiperHigh Value>"

== system DriveSystemControl/Bus Configuration (1) - Out/Simulated ECUs/Virya Controller CAN File 08082024/Telematics/RX/PDUs/TCU03/sigBrakeWiperLow/ISignal Value ==
  ISignal Value : Inport
  Term_sigBrakeWiperLow Value : Terminator
  _ISignal Value_ : BusSelector  OutputSignals=sigBrakeWiperLow Value
  wires:
  ISignal Value/1 -> _ISignal Value_/1  "ISignal Value"
  _ISignal Value_/1 -> Term_sigBrakeWiperLow Value/1  "<sigBrakeWiperLow Value>"

== system DriveSystemControl/Bus Configuration (1) - Out/Simulated ECUs/Virya Controller CAN File 08082024/Telematics/RX/PDUs/TCU03/sigCoil2DriverOpenShort/ISignal Value ==
  ISignal Value : Inport
  Term_sigCoil2DriverOpenShort Value : Terminator
  _ISignal Value_ : BusSelector  OutputSignals=sigCoil2DriverOpenShort Value
  wires:
  ISignal Value/1 -> _ISignal Value_/1  "ISignal Value"
  _ISignal Value_/1 -> Term_sigCoil2DriverOpenShort Value/1  "<sigCoil2DriverOpenShort Value>"

== system DriveSystemControl/Bus Configuration (1) - Out/Simulated ECUs/Virya Controller CAN File 08082024/Telematics/RX/PDUs/TCU03/sigCoil3DriverOpenShort/ISignal Value ==
  ISignal Value : Inport
  Term_sigCoil3DriverOpenShort Value : Terminator
  _ISignal Value_ : BusSelector  OutputSignals=sigCoil3DriverOpenShort Value
  wires:
  ISignal Value/1 -> _ISignal Value_/1  "ISignal Value"
  _ISignal Value_/1 -> Term_sigCoil3DriverOpenShort Value/1  "<sigCoil3DriverOpenShort Value>"

== system DriveSystemControl/Bus Configuration (1) - Out/Simulated ECUs/Virya Controller CAN File 08082024/Telematics/RX/PDUs/TCU03/sigCoil4DriverOpenShort/ISignal Value ==
  ISignal Value : Inport
  Term_sigCoil4DriverOpenShort Value : Terminator
  _ISignal Value_ : BusSelector  OutputSignals=sigCoil4DriverOpenShort Value
  wires:
  ISignal Value/1 -> _ISignal Value_/1  "ISignal Value"
  _ISignal Value_/1 -> Term_sigCoil4DriverOpenShort Value/1  "<sigCoil4DriverOpenShort Value>"

== system DriveSystemControl/Bus Configuration (1) - Out/Simulated ECUs/Virya Controller CAN File 08082024/Telematics/RX/PDUs/TCU03/sigControllerCommonFault/ISignal Value ==
  ISignal Value : Inport
  Term_sigControllerCommonFault Value : Terminator
  _ISignal Value_ : BusSelector  OutputSignals=sigControllerCommonFault Value
  wires:
  ISignal Value/1 -> _ISignal Value_/1  "ISignal Value"
  _ISignal Value_/1 -> Term_sigControllerCommonFault Value/1  "<sigControllerCommonFault Value>"
